simulink model "M37_Sim_Forcing_003h_expe_infra_transz_lim"  (Simulink 7.4)
settings: Solver=FixedStepDiscrete  StartTime=0.0  StopTime=inf  FixedStep=0.004  RelTol=1e-3
undefined symbols (not defined in the file or in its folder): DiscIntNeverNeededParam
libraries: simulink x39, gt_rt_lib x20, xpcutilitieslib x3, xpclib x2, dspswit3 x1
(part 3 of 4)

== system M37_Sim_Forcing_003h_expe_infra_transz_lim/Breaking_Control 20/07/15/Move_cabin/Subsystem ==
  com_or : Inport
  start_zeroing : Inport  Port=2
  connect_x : Inport  Port=3
  connect_z : Inport  Port=4
  reinit_ok : Inport  Port=5
  Display4 : Display
  Display5 : Display
  Embedded MATLAB Function3 : Stateflow chart
  Fcn : Fcn  Expr=abs(u(1))+abs(u(2))+abs(u(3))
  Logical Operator : Logic  Inputs=3  AllPortsSameDT=off  OutDataTypeMode=boolean  LogicDataType=fixdt(0, 8)  OutDataTypeStr=boolean
  Logical Operator1 : Logic  Operator=OR  AllPortsSameDT=off  OutDataTypeMode=boolean  LogicDataType=fixdt(0, 8)  OutDataTypeStr=boolean
  Logical Operator2 : Logic  Operator=NOT  AllPortsSameDT=off  OutDataTypeMode=boolean  LogicDataType=fixdt(0, 8)  OutDataTypeStr=boolean
  Logical Operator3 : Logic  AllPortsSameDT=off  OutDataTypeMode=boolean  LogicDataType=fixdt(0, 8)  OutDataTypeStr=boolean
  Logical Operator4 : Logic  AllPortsSameDT=off  OutDataTypeMode=boolean  LogicDataType=fixdt(0, 8)  OutDataTypeStr=boolean
  Logical Operator5 : Logic  Operator=OR  AllPortsSameDT=off  OutDataTypeMode=boolean  LogicDataType=fixdt(0, 8)  OutDataTypeStr=boolean
  Logical Operator6 : Logic  Operator=NOT  AllPortsSameDT=off  OutDataTypeMode=boolean  LogicDataType=fixdt(0, 8)  OutDataTypeStr=boolean
  Logical Operator7 : Logic  Inputs=4  AllPortsSameDT=off  OutDataTypeMode=boolean  LogicDataType=fixdt(0, 8)  OutDataTypeStr=boolean
  Logical Operator8 : Logic  Operator=NOT  Inputs=3  AllPortsSameDT=off  OutDataTypeMode=boolean  LogicDataType=fixdt(0, 8)  OutDataTypeStr=boolean
  Relational Operator : RelationalOperator  Operator=<=  LogicOutDataTypeMode=boolean  LogicDataType=fixdt(0, 8)  OutDataTypeStr=boolean
  Unit Delay : UnitDelay  SampleTime=-1
  gain : Constant  Value=0.004
  flag_reset : Outport  OutDataType=fixdt(1, 16)  OutScaling=2^0
  launch_reinit : Outport  Port=2  OutDataType=fixdt(1, 16)  OutScaling=2^0
  wires:
  gain/1 -> Relational Operator/2
  Logical Operator/1 -> Display4/1, flag_reset/1, Logical Operator8/1
  com_or/1 -> Embedded MATLAB Function3/1(com_or), Fcn/1
  Embedded MATLAB Function3/1(max_tilt) -> Relational Operator/1
  start_zeroing/1 -> Logical Operator3/1, Logical Operator5/1
  connect_x/1 -> Logical Operator3/2, Logical Operator6/1, Logical Operator7/3
  connect_z/1 -> Logical Operator2/1
  Logical Operator2/1 -> Logical Operator1/2
  Logical Operator3/1 -> Logical Operator1/1
  Logical Operator1/1 -> Logical Operator/2, Logical Operator7/2
  Relational Operator/1 -> Logical Operator4/1
  Logical Operator4/1 -> Logical Operator/1, Logical Operator7/1
  Logical Operator5/1 -> Logical Operator4/2
  Logical Operator6/1 -> Logical Operator5/2
  reinit_ok/1 -> Logical Operator/3
  Logical Operator7/1 -> launch_reinit/1, Display5/1
  Logical Operator8/1 -> Unit Delay/1
  Unit Delay/1 -> Logical Operator7/4

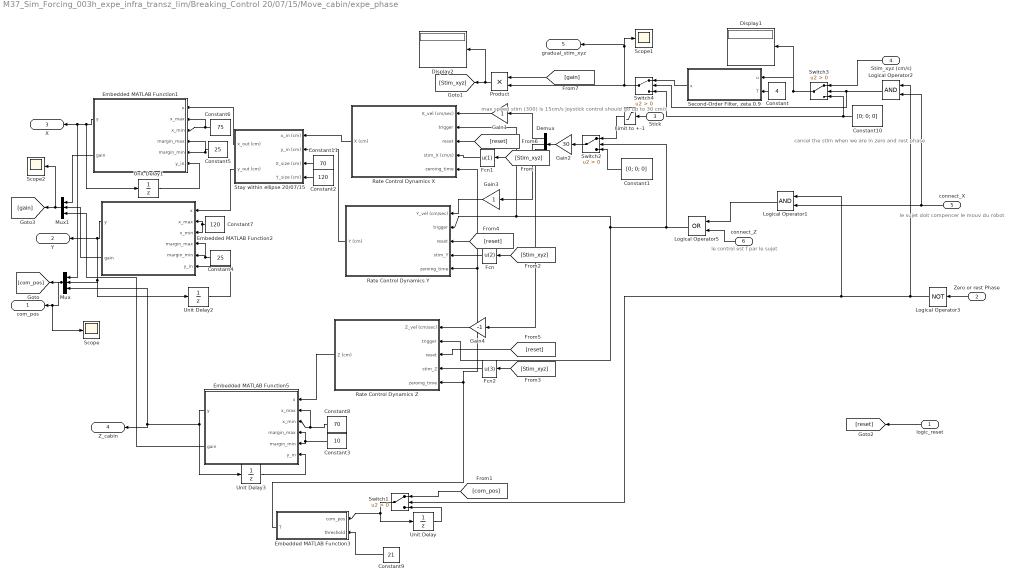
== system M37_Sim_Forcing_003h_expe_infra_transz_lim/Breaking_Control 20/07/15/Move_cabin/expe_phase ==
  note: cancel the stim when we are
      | in zero and rest phase
  note: max speed stim (300)
      | is 15cm/s
      | joystick control should go
      |  up to 30 cm/s
  note: le sujet doit compencer le mouv du robot
  note: le control est f par le sujet
  logic_reset : Inport
  Zero or rest Phase : Inport  Port=2  OutDataType=fixdt(1, 16)  OutScaling=2^0
  Stick : Inport  Port=3
  Stim_xyz (cm/s) : Inport  Port=4
  connect_X : Inport  Port=5  OutDataType=fixdt(1, 16)  OutScaling=2^0
  connect_Z : Inport  Port=6  OutDataType=fixdt(1, 16)  OutScaling=2^0
  Constant : Constant  Value=4  OutDataType=fixdt(1, 16)  OutScaling=2^0
  Constant1 : Constant  Value=[0; 0; 0]  OutDataType=fixdt(1, 16)  OutScaling=2^0
  Constant10 : Constant  Value=[0; 0; 0]  OutDataType=fixdt(1, 16)  OutScaling=2^0
  Constant11 : Constant  Value=70  OutDataType=fixdt(1, 16)  OutScaling=2^0
  Constant2 : Constant  Value=120  OutDataType=fixdt(1, 16)  OutScaling=2^0
  Constant3 : Constant  Value=10  OutDataType=fixdt(1, 16)  OutScaling=2^0
  Constant4 : Constant  Value=25  OutDataType=fixdt(1, 16)  OutScaling=2^0
  Constant5 : Constant  Value=25  OutDataType=fixdt(1, 16)  OutScaling=2^0
  Constant6 : Constant  Value=75  OutDataType=fixdt(1, 16)  OutScaling=2^0
  Constant7 : Constant  Value=120  OutDataType=fixdt(1, 16)  OutScaling=2^0
  Constant8 : Constant  Value=70  OutDataType=fixdt(1, 16)  OutScaling=2^0
  Constant9 : Constant  Value=21  OutDataType=fixdt(1, 16)  OutScaling=2^0
  Demux : Demux  Outputs=3
  Display1 : Display
  Display2 : Display
  Embedded MATLAB Function1 : Stateflow chart
  Embedded MATLAB Function2 : Stateflow chart
  Embedded MATLAB Function3 : Stateflow chart
  Embedded MATLAB Function5 : Stateflow chart
  Fcn : Fcn  Expr=u(2)
  Fcn1 : Fcn  Expr=u(1)
  Fcn2 : Fcn  Expr=u(3)
  Gain1 : Gain  ParameterDataType=fixdt(1, 16)  ParameterScaling=2^0  OutDataType=fixdt(1, 16)  OutScaling=2^0
  Gain2 : Gain  Gain=30  ParameterDataType=fixdt(1, 16)  ParameterScaling=2^0  OutDataType=fixdt(1, 16)  OutScaling=2^0
  Gain3 : Gain  ParameterDataType=fixdt(1, 16)  ParameterScaling=2^0  OutDataType=fixdt(1, 16)  OutScaling=2^0
  Gain4 : Gain  Gain=-1  ParameterDataType=fixdt(1, 16)  ParameterScaling=2^0  OutDataType=fixdt(1, 16)  OutScaling=2^0
  Limit to +-1 : Saturate  UpperLimit=1  LowerLimit=-1  OutDataType=fixdt(1, 16)  OutScaling=2^0
  Logical Operator1 : Logic  AllPortsSameDT=off  OutDataTypeMode=boolean  LogicDataType=fixdt(0, 8)  OutDataTypeStr=boolean
  Logical Operator2 : Logic  AllPortsSameDT=off  OutDataTypeMode=boolean  LogicDataType=fixdt(0, 8)  OutDataTypeStr=boolean
  Logical Operator3 : Logic  Operator=NOT  AllPortsSameDT=off  OutDataTypeMode=boolean  LogicDataType=fixdt(0, 8)  OutDataTypeStr=boolean
  Logical Operator5 : Logic  Operator=OR  AllPortsSameDT=off  OutDataTypeMode=boolean  LogicDataType=fixdt(0, 8)  OutDataTypeStr=boolean
  Mux : Mux  Inputs=3
  Mux1 : Mux  Inputs=3
  Product : Product  OutDataType=fixdt(1, 16)  OutScaling=2^0  RndMeth=Zero
  Rate Control Dynamics X : Subsystem
  Rate Control Dynamics Y : Subsystem
  Rate Control Dynamics Z : Subsystem
  Scope : Scope
      settings: TimeRange=10  YMax=65
  Scope1 : Scope
      settings: YMin=-0.5  YMax=10.5
  Scope2 : Scope
      settings: YMin=0.15  YMax=1  SaveName=ScopeData2
  "Second-Order Filter, zeta 0.9" : Subsystem
  Stay within ellipse 20/07/15 : Subsystem
  Switch{1..4} (4 alike) : Switch  Criteria=u2 > Threshold  OutDataType=fixdt(1, 16)  OutScaling=2^0
  Unit Delay : UnitDelay  X0=[0 0 0]  SampleTime=-1
  Unit Delay1 : UnitDelay  SampleTime=-1
  Unit Delay2 : UnitDelay  SampleTime=-1
  Unit Delay3 : UnitDelay  SampleTime=-1
  com_pos : Outport
  Y : Outport  Port=2
  X : Outport  Port=3
  Z_cabin : Outport  Port=4
  gradual_stim_xyz : Outport  Port=5
  wires:
  Gain2/1 -> Demux/1
  Demux/1 -> Gain1/1
  Demux/2 -> Gain3/1
  Switch2/1 -> Gain2/1
  Stick/1 -> Limit to +-1/1
  Demux/3 -> Gain4/1
  Zero or rest Phase/1 -> Logical Operator3/1
  Embedded MATLAB Function1/1(y) -> X/1, Mux/1, Unit Delay1/1
  Constant7/1 -> Embedded MATLAB Function2/2(x_max), Embedded MATLAB Function2/3(x_min)
  Embedded MATLAB Function2/1(y) -> Y/1, Mux/2, Unit Delay2/1
  Constant3/1 -> Embedded MATLAB Function5/5(margin_min), Embedded MATLAB Function5/4(margin_max)
  Constant8/1 -> Embedded MATLAB Function5/2(x_max), Embedded MATLAB Function5/3(x_min)
  Constant4/1 -> Embedded MATLAB Function2/4(margin_max), Embedded MATLAB Function2/5(margin_min)
  Constant5/1 -> Embedded MATLAB Function1/4(margin_max), Embedded MATLAB Function1/5(margin_min)
  Constant6/1 -> Embedded MATLAB Function1/3(x_min), Embedded MATLAB Function1/2(x_max)
  Constant9/1 -> Embedded MATLAB Function3/2(threshold)
  Switch1/1 -> Embedded MATLAB Function3/1(com_pos), Unit Delay/1
  Unit Delay/1 -> Switch1/3
  Embedded MATLAB Function3/1(T) -> Rate Control Dynamics X/5(zeroing_time), Rate Control Dynamics Y/5(zeroing_time), Rate Control Dynamics Z/5(zeroing_time)
  Mux/1 -> [com_pos], com_pos/1, Scope/1
  [com_pos] -> Switch1/1
  Gain3/1 -> Rate Control Dynamics Y/1(Y_vel (cm/sec))
  Gain4/1 -> Rate Control Dynamics Z/1(Z_vel (cm/sec))
  [Stim_xyz] -> Fcn/1
  [Stim_xyz] -> Fcn1/1
  [Stim_xyz] -> Fcn2/1
  Logical Operator3/1 -> Logical Operator2/1, Logical Operator1/1, Switch1/2
  Logical Operator1/1 -> Logical Operator5/1
  Constant1/1 -> Switch2/3
  Limit to +-1/1 -> Switch2/1
  connect_X/1 -> Logical Operator1/2, Logical Operator2/2
  Constant10/1 -> Switch3/3, Switch4/3
  Logical Operator2/1 -> Switch3/2, Switch4/2
  Switch3/1 -> Display1/1, "Second-Order Filter, zeta 0.9"/1(u)
  Stim_xyz (cm/s)/1 -> Switch3/1
  logic_reset/1 -> [reset]
  [reset] -> Rate Control Dynamics Y/3(reset)
  [reset] -> Rate Control Dynamics Z/3(reset)
  [reset] -> Rate Control Dynamics X/3(reset)
  Gain1/1 -> Rate Control Dynamics X/1(X_vel (cm/sec))
  Fcn1/1 -> Rate Control Dynamics X/4(stim_X (cm/s))
  Fcn/1 -> Rate Control Dynamics Y/4(stim_Y)
  Logical Operator5/1 -> Rate Control Dynamics Y/2(trigger), Rate Control Dynamics X/2(trigger), Rate Control Dynamics Z/2(trigger), Switch2/2
  connect_Z/1 -> Logical Operator5/2
  Rate Control Dynamics Z/1(Z (cm)) -> Embedded MATLAB Function5/1(x)
  Fcn2/1 -> Rate Control Dynamics Z/4(stim_Z)
  Stay within ellipse 20/07/15/1(x_out (cm)) -> Embedded MATLAB Function1/1(x)
  Stay within ellipse 20/07/15/2(y_out (cm)) -> Embedded MATLAB Function2/1(x)
  Rate Control Dynamics X/1(X (cm)) -> Stay within ellipse 20/07/15/1(x_in (cm))
  Rate Control Dynamics Y/1(Y (cm)) -> Stay within ellipse 20/07/15/2(y_in (cm))
  Constant2/1 -> Stay within ellipse 20/07/15/4(Y_size (cm))
  Constant11/1 -> Stay within ellipse 20/07/15/3(X_size (cm))
  Constant/1 -> "Second-Order Filter, zeta 0.9"/2(T)
  Switch4/1 -> gradual_stim_xyz/1, Scope1/1, Product/2
  "Second-Order Filter, zeta 0.9"/1(x) -> Switch4/1
  Unit Delay1/1 -> Embedded MATLAB Function1/6(y_in)
  Embedded MATLAB Function1/2(gain) -> Mux1/1
  Embedded MATLAB Function2/2(gain) -> Mux1/2
  Unit Delay2/1 -> Embedded MATLAB Function2/6(y_in)
  Embedded MATLAB Function5/1(y) -> Z_cabin/1, Mux/3, Unit Delay3/1
  Embedded MATLAB Function5/2(gain) -> Mux1/3
  Product/1 -> [Stim_xyz], Display2/1
  Mux1/1 -> [gain], Scope2/1
  [gain] -> Product/1
  Unit Delay3/1 -> Embedded MATLAB Function5/6(y_in)

== system M37_Sim_Forcing_003h_expe_infra_transz_lim/Breaking_Control 20/07/15/compute_offset/Smooth Displacement Second-Order Filter, zeta 0.8 ==
  Step IN Reset on  either : Inport
  T : Inport  Port=2  OutDataType=fixdt(1, 16)  OutScaling=2^0
  (zeta*T_transfer)/pi : Gain  Gain=0.8/pi  ParameterDataType=fixdt(1, 16)  ParameterScaling=2^0  OutDataType=fixdt(1, 16)  OutScaling=2^0
  4*zeta*pi : Gain  Gain=3.2*pi  ParameterDataType=fixdt(1, 16)  ParameterScaling=2^0  OutDataType=fixdt(1, 16)  OutScaling=2^0
  4*zeta*pi/T_transfer /s : DiscreteIntegrator  gainval=1  ExternalReset=either  InitialConditionSource=external  SampleTime=0.004  OutDataType=fixdt(1, 16)  OutScaling=2^0  ICPrevOutput=DiscIntNeverNeededParam  ICPrevScaledInput=DiscIntNeverNeededParam
  Discrete Derivative : simulink/Discrete/Discrete Derivative  SystemSampleTime=-1  gainval=1.0  ICPrevScaledInput=0.0  OutMin=[]  OutMax=[]  OutDataType=fixdt(1, 16)  OutScaling=2^-10  DoSatur=off
  Divide : Product  Inputs=*/  OutDataType=fixdt(1, 16)  OutScaling=2^-10
  Divide1 : Product  Inputs=*/  OutDataType=fixdt(1, 16)  OutScaling=2^-10
  For saving position  and velocity until after switchover : UnitDelay  SampleTime=-1
  Product : Product  OutDataType=fixdt(1, 16)  OutScaling=2^0  RndMeth=Zero
  Sum1 : Sum  Inputs=|+-  OutDataType=fixdt(1, 16)  OutScaling=2^0
  Sum2 : Sum  Inputs=-+|  OutDataType=fixdt(1, 16)  OutScaling=2^0
  pi/(zeta*T_transfer)/s : DiscreteIntegrator  gainval=1  ExternalReset=either  InitialConditionSource=external  SampleTime=0.004  OutDataType=fixdt(1, 16)  OutScaling=2^0  ICPrevOutput=DiscIntNeverNeededParam  ICPrevScaledInput=DiscIntNeverNeededParam
  pi/zeta : Gain  Gain=pi/0.8  ParameterDataType=fixdt(1, 16)  ParameterScaling=2^0  OutDataType=fixdt(1, 16)  OutScaling=2^0
  Out : Outport
  wires:
  Discrete Derivative/1 -> Product/2
  Product/1 -> (zeta*T_transfer)/pi/1
  Divide/1 -> 4*zeta*pi/1
  Divide1/1 -> pi/zeta/1
  pi/zeta/1 -> pi/(zeta*T_transfer)/s/1
  pi/(zeta*T_transfer)/s/1 -> Sum2/1, Out/1, For saving position  and velocity until after switchover/1
  4*zeta*pi/T_transfer /s/1 -> Divide1/1, Sum1/2
  Sum1/1 -> Divide/1
  4*zeta*pi/1 -> 4*zeta*pi/T_transfer /s/1
  T/1 -> [T]
  Step IN Reset on  either/1 -> [Step], Sum2/2
  [Step] -> 4*zeta*pi/T_transfer /s/2
  [Step] -> pi/(zeta*T_transfer)/s/2
  [T] -> Divide/2
  For saving position  and velocity until after switchover/1 -> Discrete Derivative/1, pi/(zeta*T_transfer)/s/3
  [T] -> Product/1
  (zeta*T_transfer)/pi/1 -> 4*zeta*pi/T_transfer /s/3
  [T] -> Divide1/2
  Sum2/1 -> Sum1/1

== system M37_Sim_Forcing_003h_expe_infra_transz_lim/Joint Controller (May 7, 2015)1/Forward Kinematics/KUKA2NED ==
  KUKA : Inport
  Constant : Constant  Value=[0 0 0 0 0 15.89]  OutDataType=fixdt(1, 16)  OutScaling=2^0
  Gain : Gain  Gain=[1 -1 -1 -1 -1 -1]  ParameterDataType=fixdt(1, 16)  ParameterScaling=2^0  OutDataType=fixdt(1, 16)  OutScaling=2^0
  Sum : Sum  Inputs=|++  OutDataType=fixdt(1, 16)  OutScaling=2^0
  NED : Outport
  wires:
  Gain/1 -> Sum/1
  KUKA/1 -> Gain/1
  Sum/1 -> NED/1
  Constant/1 -> Sum/2

== system M37_Sim_Forcing_003h_expe_infra_transz_lim/Joint Controller (May 7, 2015)1/Inverse Kinematics May 6, 2015/Inverse Kinematics ==
  note: (6_DOF_ACT - 6_DOF_COM) exp(-0.1t) + 6_DOF_COM
  vec : Inport
  Activate full inverse : Inport  Port=2
  6_DOF_ACT : Inport  Port=3  OutDataType=fixdt(1, 16)  OutScaling=2^0
  Demux : Demux  Outputs=[6,6]
  Discrete-Time Integrator : DiscreteIntegrator  gainval=1  ExternalReset=either  InitialConditionSource=external  SampleTime=-1  OutDataType=fixdt(1, 16)  OutScaling=2^0  ICPrevOutput=DiscIntNeverNeededParam  ICPrevScaledInput=DiscIntNeverNeededParam
  Gain : Gain  Gain=-0.1  ParameterDataType=fixdt(1, 16)  ParameterScaling=2^0  OutDataType=fixdt(1, 16)  OutScaling=2^0
  Mux : Mux  Inputs=2
  Select -6_DOF_COM : Selector  InputPortWidth=12  IndexOptions=Index vector (dialog)  Indices=[1 2 3 4 5 6]  OutputSizes=1
  Sum : Sum  Inputs=|-+  OutDataType=fixdt(1, 16)  OutScaling=2^0
  Sum1 : Sum  Inputs=|++  OutDataType=fixdt(1, 16)  OutScaling=2^0
  full inverse kin : Subsystem
  out : Outport  OutDataType=fixdt(1, 16)  OutScaling=2^0
  wires:
  vec/1 -> Select -6_DOF_COM/1, Demux/1
  full inverse kin/1(out) -> out/1
  Activate full inverse/1 -> full inverse kin/Enable, Discrete-Time Integrator/2
  Discrete-Time Integrator/1 -> Gain/1, Sum1/2
  Gain/1 -> Discrete-Time Integrator/1
  6_DOF_ACT/1 -> Sum/2
  Select -6_DOF_COM/1 -> Sum/1
  Sum/1 -> Discrete-Time Integrator/3
  Demux/2 -> Mux/2
  Demux/1 -> Sum1/1
  Sum1/1 -> Mux/1
  Mux/1 -> full inverse kin/1(vec)

== system M37_Sim_Forcing_003h_expe_infra_transz_lim/Joint Controller (May 7, 2015)1/Inverse Kinematics May 6, 2015/NED2KUKA ==
  NED : Inport
  Constant : Constant  Value=[0 0 0 0 0 15.89]  OutDataType=fixdt(1, 16)  OutScaling=2^0
  Gain : Gain  Gain=[1 -1 -1 -1 -1 -1]  ParameterDataType=fixdt(1, 16)  ParameterScaling=2^0  OutDataType=fixdt(1, 16)  OutScaling=2^0
  Sum : Sum  Inputs=|++  OutDataType=fixdt(1, 16)  OutScaling=2^0
  KUKA : Outport
  wires:
  Gain/1 -> Sum/1
  NED/1 -> Gain/1
  Sum/1 -> KUKA/1
  Constant/1 -> Sum/2

== system M37_Sim_Forcing_003h_expe_infra_transz_lim/Joint Controller (May 7, 2015)1/Inverse Kinematics May 6, 2015/Simplified Inverse Kinematics ==
  note: (A1-A6_ACT - A1-A6_COM) exp(-0.1t) + A1-A6_COM
  note: Selects and sets
      |  A1, A4,A6 to zero
  note: This version has been tested on May 6, 2015
  activate simplified : Inport  OutDataType=fixdt(1, 16)  OutScaling=2^0
  vec : Inport  Port=2  OutDataType=fixdt(1, 16)  OutScaling=2^0
  A1-A6 ACT : Selector  InputPortWidth=12  IndexOptions=Index vector (dialog)  Indices=[7 8 9 10 11 12]  OutputSizes=1
  A1-A6 COM : Subsystem
  Discrete-Time Integrator1 : DiscreteIntegrator  gainval=1  ExternalReset=either  InitialConditionSource=external  SampleTime=-1  OutDataType=fixdt(1, 16)  OutScaling=2^0  ICPrevOutput=DiscIntNeverNeededParam  ICPrevScaledInput=DiscIntNeverNeededParam
  Gain1 : Gain  Gain=-0.1  ParameterDataType=fixdt(1, 16)  ParameterScaling=2^0  OutDataType=fixdt(1, 16)  OutScaling=2^0
  Mux : Mux  Inputs=2
  N : Selector  InputPortWidth=7  IndexOptions=Index vector (dialog)  Indices=7  OutputSizes=1
  Simplified Inverse Kin : Subsystem
  Sum : Sum  Inputs=-+|  OutDataType=fixdt(1, 16)  OutScaling=2^0
  Sum1 : Sum  Inputs=++|  OutDataType=fixdt(1, 16)  OutScaling=2^0
  out : Outport  OutDataType=fixdt(1, 16)  OutScaling=2^0
  outMGI : Outport  Port=2  OutDataType=fixdt(1, 16)  OutScaling=2^0
  wires:
  vec/1 -> Simplified Inverse Kin/1(Vec), A1-A6 ACT/1
  activate simplified/1 -> Simplified Inverse Kin/Enable, Discrete-Time Integrator1/2
  Discrete-Time Integrator1/1 -> Gain1/1, Sum1/2
  Gain1/1 -> Discrete-Time Integrator1/1
  Sum1/1 -> Mux/1
  Sum/1 -> Discrete-Time Integrator1/3
  Mux/1 -> out/1
  A1-A6 ACT/1 -> Sum/2
  Simplified Inverse Kin/1(Out) -> A1-A6 COM/1(vec), N/1
  A1-A6 COM/1(A1-A6 COM) -> Sum/1, Sum1/1
  N/1 -> Mux/2
  Simplified Inverse Kin/2(Out_MGI) -> outMGI/1

== system M37_Sim_Forcing_003h_expe_infra_transz_lim/BEC (May 7, 2015)/CAN Send/If Action Subsystem1/Convert int to 4*uni8  ==
  in : Inport
  Gain{1..4} (4 alike) : Gain  ParameterDataType=fixdt(1, 16)  ParameterScaling=2^0  OutDataTypeMode=uint8  OutDataType=fixdt(1, 16)  OutScaling=2^0  OutDataTypeStr=uint8
  Mux : Mux
  Shift Arithmetic : simulink/Logic and Bit Operations/Shift Arithmetic  SystemSampleTime=-1  nBitShiftRight=8  nBinPtShiftRight=0
  Shift Arithmetic1 : simulink/Logic and Bit Operations/Shift Arithmetic  SystemSampleTime=-1  nBitShiftRight=16  nBinPtShiftRight=0
  Shift Arithmetic2 : simulink/Logic and Bit Operations/Shift Arithmetic  SystemSampleTime=-1  nBitShiftRight=24  nBinPtShiftRight=0
  out : Outport
  wires:
  in/1 -> Shift Arithmetic1/1, Gain1/1, Shift Arithmetic/1, Shift Arithmetic2/1
  Shift Arithmetic/1 -> Gain2/1
  Shift Arithmetic1/1 -> Gain3/1
  Shift Arithmetic2/1 -> Gain4/1
  Gain1/1 -> Mux/1
  Gain2/1 -> Mux/2
  Gain3/1 -> Mux/3
  Gain4/1 -> Mux/4
  Mux/1 -> out/1

== system M37_Sim_Forcing_003h_expe_infra_transz_lim/BEC (May 7, 2015)/CAN Send/If Action Subsystem1/Convert int to 4*uni8 1 ==
  in : Inport
  Gain{1..4} (4 alike) : Gain  ParameterDataType=fixdt(1, 16)  ParameterScaling=2^0  OutDataTypeMode=uint8  OutDataType=fixdt(1, 16)  OutScaling=2^0  OutDataTypeStr=uint8
  Mux : Mux
  Shift Arithmetic : simulink/Logic and Bit Operations/Shift Arithmetic  SystemSampleTime=-1  nBitShiftRight=8  nBinPtShiftRight=0
  Shift Arithmetic1 : simulink/Logic and Bit Operations/Shift Arithmetic  SystemSampleTime=-1  nBitShiftRight=16  nBinPtShiftRight=0
  Shift Arithmetic2 : simulink/Logic and Bit Operations/Shift Arithmetic  SystemSampleTime=-1  nBitShiftRight=24  nBinPtShiftRight=0
  out : Outport
  wires:
  Mux/1 -> out/1
  Gain4/1 -> Mux/4
  Gain3/1 -> Mux/3
  Gain2/1 -> Mux/2
  Gain1/1 -> Mux/1
  Shift Arithmetic2/1 -> Gain4/1
  Shift Arithmetic1/1 -> Gain3/1
  Shift Arithmetic/1 -> Gain2/1
  in/1 -> Shift Arithmetic2/1, Shift Arithmetic/1, Gain1/1, Shift Arithmetic1/1

== system M37_Sim_Forcing_003h_expe_infra_transz_lim/BEC (May 7, 2015)/CAN Send/If Action Subsystem1/Convert int to 4*uni8 2 ==
  in : Inport
  Gain{1..4} (4 alike) : Gain  ParameterDataType=fixdt(1, 16)  ParameterScaling=2^0  OutDataTypeMode=uint8  OutDataType=fixdt(1, 16)  OutScaling=2^0  OutDataTypeStr=uint8
  Mux : Mux
  Shift Arithmetic : simulink/Logic and Bit Operations/Shift Arithmetic  SystemSampleTime=-1  nBitShiftRight=8  nBinPtShiftRight=0
  Shift Arithmetic1 : simulink/Logic and Bit Operations/Shift Arithmetic  SystemSampleTime=-1  nBitShiftRight=16  nBinPtShiftRight=0
  Shift Arithmetic2 : simulink/Logic and Bit Operations/Shift Arithmetic  SystemSampleTime=-1  nBitShiftRight=24  nBinPtShiftRight=0
  out : Outport
  wires:
  Mux/1 -> out/1
  Gain4/1 -> Mux/4
  Gain3/1 -> Mux/3
  Gain2/1 -> Mux/2
  Gain1/1 -> Mux/1
  Shift Arithmetic2/1 -> Gain4/1
  Shift Arithmetic1/1 -> Gain3/1
  Shift Arithmetic/1 -> Gain2/1
  in/1 -> Shift Arithmetic2/1, Shift Arithmetic/1, Gain1/1, Shift Arithmetic1/1

== system M37_Sim_Forcing_003h_expe_infra_transz_lim/BEC (May 7, 2015)/CAN Send/If Action Subsystem1/Convert int to 4*uni8 3 ==
  in : Inport
  Gain{1..4} (4 alike) : Gain  ParameterDataType=fixdt(1, 16)  ParameterScaling=2^0  OutDataTypeMode=uint8  OutDataType=fixdt(1, 16)  OutScaling=2^0  OutDataTypeStr=uint8
  Mux : Mux
  Shift Arithmetic : simulink/Logic and Bit Operations/Shift Arithmetic  SystemSampleTime=-1  nBitShiftRight=8  nBinPtShiftRight=0
  Shift Arithmetic1 : simulink/Logic and Bit Operations/Shift Arithmetic  SystemSampleTime=-1  nBitShiftRight=16  nBinPtShiftRight=0
  Shift Arithmetic2 : simulink/Logic and Bit Operations/Shift Arithmetic  SystemSampleTime=-1  nBitShiftRight=24  nBinPtShiftRight=0
  out : Outport
  wires:
  in/1 -> Shift Arithmetic1/1, Gain1/1, Shift Arithmetic/1, Shift Arithmetic2/1
  Shift Arithmetic/1 -> Gain2/1
  Shift Arithmetic1/1 -> Gain3/1
  Shift Arithmetic2/1 -> Gain4/1
  Gain1/1 -> Mux/1
  Gain2/1 -> Mux/2
  Gain3/1 -> Mux/3
  Gain4/1 -> Mux/4
  Mux/1 -> out/1

== system M37_Sim_Forcing_003h_expe_infra_transz_lim/BEC (May 7, 2015)/CAN Send/If Action Subsystem1/Convert int to 4*uni8 4 ==
  in : Inport
  Gain{1..4} (4 alike) : Gain  ParameterDataType=fixdt(1, 16)  ParameterScaling=2^0  OutDataTypeMode=uint8  OutDataType=fixdt(1, 16)  OutScaling=2^0  OutDataTypeStr=uint8
  Mux : Mux
  Shift Arithmetic : simulink/Logic and Bit Operations/Shift Arithmetic  SystemSampleTime=-1  nBitShiftRight=8  nBinPtShiftRight=0
  Shift Arithmetic1 : simulink/Logic and Bit Operations/Shift Arithmetic  SystemSampleTime=-1  nBitShiftRight=16  nBinPtShiftRight=0
  Shift Arithmetic2 : simulink/Logic and Bit Operations/Shift Arithmetic  SystemSampleTime=-1  nBitShiftRight=24  nBinPtShiftRight=0
  out : Outport
  wires:
  in/1 -> Shift Arithmetic1/1, Gain1/1, Shift Arithmetic/1, Shift Arithmetic2/1
  Shift Arithmetic/1 -> Gain2/1
  Shift Arithmetic1/1 -> Gain3/1
  Shift Arithmetic2/1 -> Gain4/1
  Gain1/1 -> Mux/1
  Gain2/1 -> Mux/2
  Gain3/1 -> Mux/3
  Gain4/1 -> Mux/4
  Mux/1 -> out/1

== system M37_Sim_Forcing_003h_expe_infra_transz_lim/BEC (May 7, 2015)/CAN Send/If Action Subsystem1/Convert int to 4*uni8 5 ==
  in : Inport
  Gain{1..4} (4 alike) : Gain  ParameterDataType=fixdt(1, 16)  ParameterScaling=2^0  OutDataTypeMode=uint8  OutDataType=fixdt(1, 16)  OutScaling=2^0  OutDataTypeStr=uint8
  Mux : Mux
  Shift Arithmetic : simulink/Logic and Bit Operations/Shift Arithmetic  SystemSampleTime=-1  nBitShiftRight=8  nBinPtShiftRight=0
  Shift Arithmetic1 : simulink/Logic and Bit Operations/Shift Arithmetic  SystemSampleTime=-1  nBitShiftRight=16  nBinPtShiftRight=0
  Shift Arithmetic2 : simulink/Logic and Bit Operations/Shift Arithmetic  SystemSampleTime=-1  nBitShiftRight=24  nBinPtShiftRight=0
  out : Outport
  wires:
  Mux/1 -> out/1
  Gain4/1 -> Mux/4
  Gain3/1 -> Mux/3
  Gain2/1 -> Mux/2
  Gain1/1 -> Mux/1
  Shift Arithmetic2/1 -> Gain4/1
  Shift Arithmetic1/1 -> Gain3/1
  Shift Arithmetic/1 -> Gain2/1
  in/1 -> Shift Arithmetic2/1, Shift Arithmetic/1, Gain1/1, Shift Arithmetic1/1

== system M37_Sim_Forcing_003h_expe_infra_transz_lim/BEC (May 7, 2015)/Software limit switches/Subsystem/If Action Subsystem ==
  dif : Inport  OutDataType=fixdt(1, 16)  OutScaling=2^0
  Inc : Inport  Port=2  OutDataType=fixdt(1, 16)  OutScaling=2^0
  Action Port : ActionPort  ActionType=then
  PSEA2 : Constant  Value=0  OutDataType=fixdt(1, 16)  OutScaling=2^0
  Switch : Switch  Criteria=u2 > Threshold  Threshold=1  OutDataType=fixdt(1, 16)  OutScaling=2^0
  Out1 : Outport  OutDataType=fixdt(1, 16)  OutScaling=2^0
  wires:
  PSEA2/1 -> Switch/3
  Switch/1 -> Out1/1
  Inc/1 -> Switch/1
  dif/1 -> Switch/2

== system M37_Sim_Forcing_003h_expe_infra_transz_lim/BEC (May 7, 2015)/Software limit switches/Subsystem/If Action Subsystem1 ==
  Inc : Inport  OutDataType=fixdt(1, 16)  OutScaling=2^0
  dif : Inport  Port=2  OutDataType=fixdt(1, 16)  OutScaling=2^0
  Action Port : ActionPort  ActionType=else
  PSEA2 : Constant  Value=0  OutDataType=fixdt(1, 16)  OutScaling=2^0
  Switch : Switch  Threshold=1  OutDataType=fixdt(1, 16)  OutScaling=2^0
  Out1 : Outport  OutDataType=fixdt(1, 16)  OutScaling=2^0
  wires:
  dif/1 -> Switch/2
  Inc/1 -> Switch/1
  Switch/1 -> Out1/1
  PSEA2/1 -> Switch/3

== system M37_Sim_Forcing_003h_expe_infra_transz_lim/BEC (May 7, 2015)/Software limit switches/Subsystem1/If Action Subsystem ==
  dif : Inport  OutDataType=fixdt(1, 16)  OutScaling=2^0
  Inc : Inport  Port=2  OutDataType=fixdt(1, 16)  OutScaling=2^0
  Action Port : ActionPort  ActionType=then
  PSEA2 : Constant  Value=0  OutDataType=fixdt(1, 16)  OutScaling=2^0
  Switch : Switch  Threshold=1  OutDataType=fixdt(1, 16)  OutScaling=2^0
  Out1 : Outport  OutDataType=fixdt(1, 16)  OutScaling=2^0
  wires:
  dif/1 -> Switch/2
  Inc/1 -> Switch/1
  Switch/1 -> Out1/1
  PSEA2/1 -> Switch/3

== system M37_Sim_Forcing_003h_expe_infra_transz_lim/BEC (May 7, 2015)/Software limit switches/Subsystem1/If Action Subsystem1 ==
  Inc : Inport  OutDataType=fixdt(1, 16)  OutScaling=2^0
  dif : Inport  Port=2  OutDataType=fixdt(1, 16)  OutScaling=2^0
  Action Port : ActionPort  ActionType=else
  PSEA2 : Constant  Value=0  OutDataType=fixdt(1, 16)  OutScaling=2^0
  Switch : Switch  Threshold=1  OutDataType=fixdt(1, 16)  OutScaling=2^0
  Out1 : Outport  OutDataType=fixdt(1, 16)  OutScaling=2^0
  wires:
  PSEA2/1 -> Switch/3
  Switch/1 -> Out1/1
  Inc/1 -> Switch/1
  dif/1 -> Switch/2

== system M37_Sim_Forcing_003h_expe_infra_transz_lim/BEC (May 7, 2015)/Software limit switches/Subsystem2/If Action Subsystem ==
  dif : Inport  OutDataType=fixdt(1, 16)  OutScaling=2^0
  Inc : Inport  Port=2  OutDataType=fixdt(1, 16)  OutScaling=2^0
  Action Port : ActionPort  ActionType=then
  PSEA2 : Constant  Value=0  OutDataType=fixdt(1, 16)  OutScaling=2^0
  Switch : Switch  Threshold=1  OutDataType=fixdt(1, 16)  OutScaling=2^0
  Out1 : Outport  OutDataType=fixdt(1, 16)  OutScaling=2^0
  wires:
  PSEA2/1 -> Switch/3
  Switch/1 -> Out1/1
  Inc/1 -> Switch/1
  dif/1 -> Switch/2

== system M37_Sim_Forcing_003h_expe_infra_transz_lim/BEC (May 7, 2015)/Software limit switches/Subsystem2/If Action Subsystem1 ==
  Inc : Inport  OutDataType=fixdt(1, 16)  OutScaling=2^0
  dif : Inport  Port=2  OutDataType=fixdt(1, 16)  OutScaling=2^0
  Action Port : ActionPort  ActionType=else
  PSEA2 : Constant  Value=0  OutDataType=fixdt(1, 16)  OutScaling=2^0
  Switch : Switch  Threshold=1  OutDataType=fixdt(1, 16)  OutScaling=2^0
  Out1 : Outport  OutDataType=fixdt(1, 16)  OutScaling=2^0
  wires:
  dif/1 -> Switch/2
  Inc/1 -> Switch/1
  Switch/1 -> Out1/1
  PSEA2/1 -> Switch/3

== system M37_Sim_Forcing_003h_expe_infra_transz_lim/BEC (May 7, 2015)/Software limit switches/Subsystem3/If Action Subsystem ==
  dif : Inport  OutDataType=fixdt(1, 16)  OutScaling=2^0
  Inc : Inport  Port=2  OutDataType=fixdt(1, 16)  OutScaling=2^0
  Action Port : ActionPort  ActionType=then
  PSEA2 : Constant  Value=0  OutDataType=fixdt(1, 16)  OutScaling=2^0
  Switch : Switch  Threshold=1  OutDataType=fixdt(1, 16)  OutScaling=2^0
  Out1 : Outport  OutDataType=fixdt(1, 16)  OutScaling=2^0
  wires:
  dif/1 -> Switch/2
  Inc/1 -> Switch/1
  Switch/1 -> Out1/1
  PSEA2/1 -> Switch/3

== system M37_Sim_Forcing_003h_expe_infra_transz_lim/BEC (May 7, 2015)/Software limit switches/Subsystem3/If Action Subsystem1 ==
  Inc : Inport  OutDataType=fixdt(1, 16)  OutScaling=2^0
  dif : Inport  Port=2  OutDataType=fixdt(1, 16)  OutScaling=2^0
  Action Port : ActionPort  ActionType=else
  PSEA2 : Constant  Value=0  OutDataType=fixdt(1, 16)  OutScaling=2^0
  Switch : Switch  Threshold=1  OutDataType=fixdt(1, 16)  OutScaling=2^0
  Out1 : Outport  OutDataType=fixdt(1, 16)  OutScaling=2^0
  wires:
  PSEA2/1 -> Switch/3
  Switch/1 -> Out1/1
  Inc/1 -> Switch/1
  dif/1 -> Switch/2

== system M37_Sim_Forcing_003h_expe_infra_transz_lim/BEC (May 7, 2015)/Software limit switches/Subsystem4/If Action Subsystem ==
  dif : Inport  OutDataType=fixdt(1, 16)  OutScaling=2^0
  Inc : Inport  Port=2  OutDataType=fixdt(1, 16)  OutScaling=2^0
  Action Port : ActionPort  ActionType=then
  PSEA2 : Constant  Value=0  OutDataType=fixdt(1, 16)  OutScaling=2^0
  Switch : Switch  Threshold=1  OutDataType=fixdt(1, 16)  OutScaling=2^0
  Out1 : Outport  OutDataType=fixdt(1, 16)  OutScaling=2^0
  wires:
  PSEA2/1 -> Switch/3
  Switch/1 -> Out1/1
  Inc/1 -> Switch/1
  dif/1 -> Switch/2

== system M37_Sim_Forcing_003h_expe_infra_transz_lim/BEC (May 7, 2015)/Software limit switches/Subsystem4/If Action Subsystem1 ==
  Inc : Inport  OutDataType=fixdt(1, 16)  OutScaling=2^0
  dif : Inport  Port=2  OutDataType=fixdt(1, 16)  OutScaling=2^0
  Action Port : ActionPort  ActionType=else
  PSEA2 : Constant  Value=0  OutDataType=fixdt(1, 16)  OutScaling=2^0
  Switch : Switch  Threshold=1  OutDataType=fixdt(1, 16)  OutScaling=2^0
  Out1 : Outport  OutDataType=fixdt(1, 16)  OutScaling=2^0
  wires:
  dif/1 -> Switch/2
  Inc/1 -> Switch/1
  Switch/1 -> Out1/1
  PSEA2/1 -> Switch/3

== system M37_Sim_Forcing_003h_expe_infra_transz_lim/BEC (May 7, 2015)/Software limit switches/Subsystem5/If Action Subsystem ==
  dif : Inport  OutDataType=fixdt(1, 16)  OutScaling=2^0
  Inc : Inport  Port=2  OutDataType=fixdt(1, 16)  OutScaling=2^0
  Action Port : ActionPort  ActionType=then
  PSEA2 : Constant  Value=0  OutDataType=fixdt(1, 16)  OutScaling=2^0
  Switch : Switch  Threshold=1  OutDataType=fixdt(1, 16)  OutScaling=2^0
  Out1 : Outport  OutDataType=fixdt(1, 16)  OutScaling=2^0
  wires:
  dif/1 -> Switch/2
  Inc/1 -> Switch/1
  Switch/1 -> Out1/1
  PSEA2/1 -> Switch/3

== system M37_Sim_Forcing_003h_expe_infra_transz_lim/BEC (May 7, 2015)/Software limit switches/Subsystem5/If Action Subsystem1 ==
  Inc : Inport  OutDataType=fixdt(1, 16)  OutScaling=2^0
  dif : Inport  Port=2  OutDataType=fixdt(1, 16)  OutScaling=2^0
  Action Port : ActionPort  ActionType=else
  PSEA2 : Constant  Value=0  OutDataType=fixdt(1, 16)  OutScaling=2^0
  Switch : Switch  Threshold=1  OutDataType=fixdt(1, 16)  OutScaling=2^0
  Out1 : Outport  OutDataType=fixdt(1, 16)  OutScaling=2^0
  wires:
  PSEA2/1 -> Switch/3
  Switch/1 -> Out1/1
  Inc/1 -> Switch/1
  dif/1 -> Switch/2

== system M37_Sim_Forcing_003h_expe_infra_transz_lim/Breaking_Control 20/07/15/Ellipse motion/Phase Shifted Sine 17th 1/Smooth Displacement Second-Order Filter, zeta 0.8 ==
  Step IN Reset on  either : Inport
  T : Inport  Port=2  OutDataType=fixdt(1, 16)  OutScaling=2^0
  (zeta*T_transfer)/pi : Gain  Gain=0.8/pi  ParameterDataType=fixdt(1, 16)  ParameterScaling=2^0  OutDataType=fixdt(1, 16)  OutScaling=2^0
  4*zeta*pi : Gain  Gain=3.2*pi  ParameterDataType=fixdt(1, 16)  ParameterScaling=2^0  OutDataType=fixdt(1, 16)  OutScaling=2^0
  4*zeta*pi/T_transfer /s : DiscreteIntegrator  gainval=1  ExternalReset=either  InitialConditionSource=external  SampleTime=-1  OutDataType=fixdt(1, 16)  OutScaling=2^0  ICPrevOutput=DiscIntNeverNeededParam  ICPrevScaledInput=DiscIntNeverNeededParam
  Data Type Conversion4 : DataTypeConversion  OutDataTypeMode=single  OutDataType=fixdt(1, 16)  OutScaling=2^0  OutDataTypeStr=single
  Discrete Derivative : simulink/Discrete/Discrete Derivative  SystemSampleTime=-1  gainval=1.0  ICPrevScaledInput=0.0  OutMin=[]  OutMax=[]  OutDataType=fixdt(1, 16)  OutScaling=2^-10  DoSatur=off
  Divide : Product  Inputs=*/  OutDataType=fixdt(1, 16)  OutScaling=2^-10
  Divide1 : Product  Inputs=*/  OutDataType=fixdt(1, 16)  OutScaling=2^-10
  For saving position  and velocity until after switchover : UnitDelay  SampleTime=-1
  Product : Product  OutDataType=fixdt(1, 16)  OutScaling=2^0  RndMeth=Zero
  Sum1 : Sum  Inputs=|+-  OutDataType=fixdt(1, 16)  OutScaling=2^0
  Sum2 : Sum  Inputs=-+|  OutDataType=fixdt(1, 16)  OutScaling=2^0
  pi/(zeta*T_transfer)/s : DiscreteIntegrator  gainval=1  ExternalReset=either  InitialConditionSource=external  SampleTime=-1  OutDataType=fixdt(1, 16)  OutScaling=2^0  ICPrevOutput=DiscIntNeverNeededParam  ICPrevScaledInput=DiscIntNeverNeededParam
  pi/zeta : Gain  Gain=pi/0.8  ParameterDataType=fixdt(1, 16)  ParameterScaling=2^0  OutDataType=fixdt(1, 16)  OutScaling=2^0
  Out : Outport
  wires:
  Discrete Derivative/1 -> Product/2
  Product/1 -> (zeta*T_transfer)/pi/1
  Divide/1 -> 4*zeta*pi/1
  Divide1/1 -> pi/zeta/1
  pi/zeta/1 -> pi/(zeta*T_transfer)/s/1
  pi/(zeta*T_transfer)/s/1 -> Sum2/1, For saving position  and velocity until after switchover/1, Data Type Conversion4/1
  4*zeta*pi/T_transfer /s/1 -> Divide1/1, Sum1/2
  Sum1/1 -> Divide/1
  4*zeta*pi/1 -> 4*zeta*pi/T_transfer /s/1
  T/1 -> [T]
  Step IN Reset on  either/1 -> [Step], Sum2/2
  [Step] -> 4*zeta*pi/T_transfer /s/2
  [Step] -> pi/(zeta*T_transfer)/s/2
  [T] -> Divide/2
  For saving position  and velocity until after switchover/1 -> Discrete Derivative/1, pi/(zeta*T_transfer)/s/3
  [T] -> Product/1
  (zeta*T_transfer)/pi/1 -> 4*zeta*pi/T_transfer /s/3
  [T] -> Divide1/2
  Sum2/1 -> Sum1/1
  Data Type Conversion4/1 -> Out/1

== system M37_Sim_Forcing_003h_expe_infra_transz_lim/Breaking_Control 20/07/15/Ellipse motion/Phase Shifted Sine 17th 2/Smooth Displacement Second-Order Filter, zeta 0.8 ==
  Step IN Reset on  either : Inport
  T : Inport  Port=2  OutDataType=fixdt(1, 16)  OutScaling=2^0
  (zeta*T_transfer)/pi : Gain  Gain=0.8/pi  ParameterDataType=fixdt(1, 16)  ParameterScaling=2^0  OutDataType=fixdt(1, 16)  OutScaling=2^0
  4*zeta*pi : Gain  Gain=3.2*pi  ParameterDataType=fixdt(1, 16)  ParameterScaling=2^0  OutDataType=fixdt(1, 16)  OutScaling=2^0
  4*zeta*pi/T_transfer /s : DiscreteIntegrator  gainval=1  ExternalReset=either  InitialConditionSource=external  SampleTime=-1  OutDataType=fixdt(1, 16)  OutScaling=2^0  ICPrevOutput=DiscIntNeverNeededParam  ICPrevScaledInput=DiscIntNeverNeededParam
  Data Type Conversion4 : DataTypeConversion  OutDataTypeMode=single  OutDataType=fixdt(1, 16)  OutScaling=2^0  OutDataTypeStr=single
  Discrete Derivative : simulink/Discrete/Discrete Derivative  SystemSampleTime=-1  gainval=1.0  ICPrevScaledInput=0.0  OutMin=[]  OutMax=[]  OutDataType=fixdt(1, 16)  OutScaling=2^-10  DoSatur=off
  Divide : Product  Inputs=*/  OutDataType=fixdt(1, 16)  OutScaling=2^-10
  Divide1 : Product  Inputs=*/  OutDataType=fixdt(1, 16)  OutScaling=2^-10
  For saving position  and velocity until after switchover : UnitDelay  SampleTime=-1
  Product : Product  OutDataType=fixdt(1, 16)  OutScaling=2^0  RndMeth=Zero
  Sum1 : Sum  Inputs=|+-  OutDataType=fixdt(1, 16)  OutScaling=2^0
  Sum2 : Sum  Inputs=-+|  OutDataType=fixdt(1, 16)  OutScaling=2^0
  pi/(zeta*T_transfer)/s : DiscreteIntegrator  gainval=1  ExternalReset=either  InitialConditionSource=external  SampleTime=-1  OutDataType=fixdt(1, 16)  OutScaling=2^0  ICPrevOutput=DiscIntNeverNeededParam  ICPrevScaledInput=DiscIntNeverNeededParam
  pi/zeta : Gain  Gain=pi/0.8  ParameterDataType=fixdt(1, 16)  ParameterScaling=2^0  OutDataType=fixdt(1, 16)  OutScaling=2^0
  Out : Outport
  wires:
  Discrete Derivative/1 -> Product/2
  Product/1 -> (zeta*T_transfer)/pi/1
  Divide/1 -> 4*zeta*pi/1
  Divide1/1 -> pi/zeta/1
  pi/zeta/1 -> pi/(zeta*T_transfer)/s/1
  pi/(zeta*T_transfer)/s/1 -> Sum2/1, For saving position  and velocity until after switchover/1, Data Type Conversion4/1
  4*zeta*pi/T_transfer /s/1 -> Divide1/1, Sum1/2
  Sum1/1 -> Divide/1
  4*zeta*pi/1 -> 4*zeta*pi/T_transfer /s/1
  T/1 -> [T]
  Step IN Reset on  either/1 -> [Step], Sum2/2
  [Step] -> 4*zeta*pi/T_transfer /s/2
  [Step] -> pi/(zeta*T_transfer)/s/2
  [T] -> Divide/2
  For saving position  and velocity until after switchover/1 -> Discrete Derivative/1, pi/(zeta*T_transfer)/s/3
  [T] -> Product/1
  (zeta*T_transfer)/pi/1 -> 4*zeta*pi/T_transfer /s/3
  [T] -> Divide1/2
  Sum2/1 -> Sum1/1
  Data Type Conversion4/1 -> Out/1

== system M37_Sim_Forcing_003h_expe_infra_transz_lim/Breaking_Control 20/07/15/Ellipse motion/Phase Shifted Sine 17th 2015/Smooth Displacement Second-Order Filter, zeta 0.8 ==
  note: s
  note: m
  note: y
  note: p
  note: t
  Step IN Reset on  either : Inport
  T : Inport  Port=2  OutDataType=fixdt(1, 16)  OutScaling=2^0
  (zeta*T_transfer)/pi : Gain  Gain=0.8/pi  ParameterDataType=fixdt(1, 16)  ParameterScaling=2^0  OutDataType=fixdt(1, 16)  OutScaling=2^0
  4*zeta*pi : Gain  Gain=3.2*pi  ParameterDataType=fixdt(1, 16)  ParameterScaling=2^0  OutDataType=fixdt(1, 16)  OutScaling=2^0
  4*zeta*pi/T_transfer /s : DiscreteIntegrator  gainval=1  ExternalReset=either  InitialConditionSource=external  SampleTime=-1  OutDataType=fixdt(1, 16)  OutScaling=2^0  ICPrevOutput=DiscIntNeverNeededParam  ICPrevScaledInput=DiscIntNeverNeededParam
  Data Type Conversion4 : DataTypeConversion  OutDataTypeMode=single  OutDataType=fixdt(1, 16)  OutScaling=2^0  OutDataTypeStr=single
  Discrete Derivative : simulink/Discrete/Discrete Derivative  SystemSampleTime=-1  gainval=1.0  ICPrevScaledInput=0.0  OutMin=[]  OutMax=[]  OutDataType=fixdt(1, 16)  OutScaling=2^-10  DoSatur=off
  Divide : Product  Inputs=*/  OutDataType=fixdt(1, 16)  OutScaling=2^-10
  Divide1 : Product  Inputs=*/  OutDataType=fixdt(1, 16)  OutScaling=2^-10
  For saving position  and velocity until after switchover : UnitDelay  SampleTime=-1
  Product : Product  OutDataType=fixdt(1, 16)  OutScaling=2^0  RndMeth=Zero
  Sum1 : Sum  Inputs=|+-  OutDataType=fixdt(1, 16)  OutScaling=2^0
  Sum2 : Sum  Inputs=-+|  OutDataType=fixdt(1, 16)  OutScaling=2^0
  pi/(zeta*T_transfer)/s : DiscreteIntegrator  gainval=1  ExternalReset=either  InitialConditionSource=external  SampleTime=-1  OutDataType=fixdt(1, 16)  OutScaling=2^0  ICPrevOutput=DiscIntNeverNeededParam  ICPrevScaledInput=DiscIntNeverNeededParam
  pi/zeta : Gain  Gain=pi/0.8  ParameterDataType=fixdt(1, 16)  ParameterScaling=2^0  OutDataType=fixdt(1, 16)  OutScaling=2^0
  Out : Outport
  wires:
  Discrete Derivative/1 -> Product/2
  Product/1 -> (zeta*T_transfer)/pi/1
  Divide/1 -> 4*zeta*pi/1
  Divide1/1 -> pi/zeta/1
  pi/zeta/1 -> pi/(zeta*T_transfer)/s/1
  pi/(zeta*T_transfer)/s/1 -> Sum2/1, For saving position  and velocity until after switchover/1, Data Type Conversion4/1
  4*zeta*pi/T_transfer /s/1 -> Divide1/1, Sum1/2
  Sum1/1 -> Divide/1
  4*zeta*pi/1 -> 4*zeta*pi/T_transfer /s/1
  T/1 -> [T]
  Step IN Reset on  either/1 -> [Step], Sum2/2
  [Step] -> 4*zeta*pi/T_transfer /s/2
  [Step] -> pi/(zeta*T_transfer)/s/2
  [T] -> Divide/2
  For saving position  and velocity until after switchover/1 -> Discrete Derivative/1, pi/(zeta*T_transfer)/s/3
  [T] -> Product/1
  (zeta*T_transfer)/pi/1 -> 4*zeta*pi/T_transfer /s/3
  [T] -> Divide1/2
  Sum2/1 -> Sum1/1
  Data Type Conversion4/1 -> Out/1

== system M37_Sim_Forcing_003h_expe_infra_transz_lim/Breaking_Control 20/07/15/Move_cabin/expe_phase/Rate Control Dynamics X ==
  X_vel (cm/sec) : Inport
  trigger : Inport  Port=2
  reset : Inport  Port=3
  stim_X (cm/s) : Inport  Port=4
  zeroing_time : Inport  Port=5
  Constant : Constant  Value=0.2  OutDataType=fixdt(1, 16)  OutScaling=2^0
  Constant1 : Constant  Value=15  OutDataType=fixdt(1, 16)  OutScaling=2^0
  Constant2 : Constant  Value=0.1  OutDataType=fixdt(1, 16)  OutScaling=2^0
  Discrete-Time Integrator1 : DiscreteIntegrator  ExternalReset=either  SampleTime=0.004  OutDataType=fixdt(1, 16)  OutScaling=2^0  ICPrevOutput=DiscIntNeverNeededParam  ICPrevScaledInput=DiscIntNeverNeededParam
  Display1 : Display
  Display2 : Display
  Display4 : Display
  Product : Product  OutDataType=fixdt(1, 16)  OutScaling=2^0  RndMeth=Zero
  "Second-Order Filter, zeta 0.8" : Subsystem
  "Smooth Displacement Second-Order Filter, zeta 0.8" : Subsystem
  Sum2 : Sum  Inputs=++|  OutDataType=fixdt(1, 16)  OutScaling=2^0
  Switch : Switch  Criteria=u2 > Threshold  OutDataType=fixdt(1, 16)  OutScaling=2^0
  X (cm) : Outport
  wires:
  "Second-Order Filter, zeta 0.8"/1(x) -> Discrete-Time Integrator1/1
  Constant/1 -> "Second-Order Filter, zeta 0.8"/2(T)
  Discrete-Time Integrator1/1 -> Product/1, Display2/1
  Product/1 -> X (cm)/1
  "Smooth Displacement Second-Order Filter, zeta 0.8"/1(Out) -> Product/2, Display4/1
  reset/1 -> Discrete-Time Integrator1/2
  trigger/1 -> "Smooth Displacement Second-Order Filter, zeta 0.8"/1(Step IN Reset on  either), Switch/2
  Switch/1 -> "Smooth Displacement Second-Order Filter, zeta 0.8"/2(T)
  Constant2/1 -> Switch/1
  stim_X (cm/s)/1 -> Sum2/1, Display1/1
  zeroing_time/1 -> Switch/3
  Sum2/1 -> "Second-Order Filter, zeta 0.8"/1(u)
  X_vel (cm/sec)/1 -> Sum2/2

== system M37_Sim_Forcing_003h_expe_infra_transz_lim/Breaking_Control 20/07/15/Move_cabin/expe_phase/Rate Control Dynamics Y ==
  Y_vel (cm/sec) : Inport
  trigger : Inport  Port=2
  reset : Inport  Port=3
  stim_Y : Inport  Port=4
  zeroing_time : Inport  Port=5
  Constant : Constant  Value=0.2  OutDataType=fixdt(1, 16)  OutScaling=2^0
  Constant1 : Constant  Value=15  OutDataType=fixdt(1, 16)  OutScaling=2^0
  Constant3 : Constant  Value=0.1  OutDataType=fixdt(1, 16)  OutScaling=2^0
  Discrete-Time Integrator1 : DiscreteIntegrator  ExternalReset=either  SampleTime=0.004  OutDataType=fixdt(1, 16)  OutScaling=2^0  ICPrevOutput=DiscIntNeverNeededParam  ICPrevScaledInput=DiscIntNeverNeededParam
  Display4 : Display
  Product : Product  OutDataType=fixdt(1, 16)  OutScaling=2^0  RndMeth=Zero
  "Second-Order Filter, zeta 0.8" : Subsystem
  "Smooth Displacement Second-Order Filter, zeta 0.8" : Subsystem
  Sum2 : Sum  Inputs=++|  OutDataType=fixdt(1, 16)  OutScaling=2^0
  Switch : Switch  Criteria=u2 > Threshold  OutDataType=fixdt(1, 16)  OutScaling=2^0
  Y (cm) : Outport
  wires:
  "Second-Order Filter, zeta 0.8"/1(x) -> Discrete-Time Integrator1/1
  Constant/1 -> "Second-Order Filter, zeta 0.8"/2(T)
  Discrete-Time Integrator1/1 -> Product/1
  Product/1 -> Y (cm)/1
  "Smooth Displacement Second-Order Filter, zeta 0.8"/1(Out) -> Product/2, Display4/1
  trigger/1 -> "Smooth Displacement Second-Order Filter, zeta 0.8"/1(Step IN Reset on  either), Switch/2
  reset/1 -> Discrete-Time Integrator1/2
  Constant3/1 -> Switch/1
  Switch/1 -> "Smooth Displacement Second-Order Filter, zeta 0.8"/2(T)
  stim_Y/1 -> Sum2/1
  zeroing_time/1 -> Switch/3
  Sum2/1 -> "Second-Order Filter, zeta 0.8"/1(u)
  Y_vel (cm/sec)/1 -> Sum2/2

== system M37_Sim_Forcing_003h_expe_infra_transz_lim/Breaking_Control 20/07/15/Move_cabin/expe_phase/Rate Control Dynamics Z ==
  Z_vel (cm/sec) : Inport
  trigger : Inport  Port=2
  reset : Inport  Port=3
  stim_Z : Inport  Port=4
  zeroing_time : Inport  Port=5
  Constant : Constant  Value=0.2  OutDataType=fixdt(1, 16)  OutScaling=2^0
  Constant1 : Constant  Value=15  OutDataType=fixdt(1, 16)  OutScaling=2^0
  Constant3 : Constant  Value=0.1  OutDataType=fixdt(1, 16)  OutScaling=2^0
  Discrete-Time Integrator1 : DiscreteIntegrator  ExternalReset=either  SampleTime=0.004  OutDataType=fixdt(1, 16)  OutScaling=2^0  ICPrevOutput=DiscIntNeverNeededParam  ICPrevScaledInput=DiscIntNeverNeededParam
  Display4 : Display
  Product : Product  OutDataType=fixdt(1, 16)  OutScaling=2^0  RndMeth=Zero
  "Second-Order Filter, zeta 0.8" : Subsystem
  "Smooth Displacement Second-Order Filter, zeta 0.8" : Subsystem
  Sum2 : Sum  Inputs=++|  OutDataType=fixdt(1, 16)  OutScaling=2^0
  Switch : Switch  Criteria=u2 > Threshold  OutDataType=fixdt(1, 16)  OutScaling=2^0
  Z (cm) : Outport
  wires:
  "Second-Order Filter, zeta 0.8"/1(x) -> Discrete-Time Integrator1/1
  Constant/1 -> "Second-Order Filter, zeta 0.8"/2(T)
  Discrete-Time Integrator1/1 -> Product/1
  Product/1 -> Z (cm)/1
  "Smooth Displacement Second-Order Filter, zeta 0.8"/1(Out) -> Product/2, Display4/1
  trigger/1 -> "Smooth Displacement Second-Order Filter, zeta 0.8"/1(Step IN Reset on  either), Switch/2
  reset/1 -> Discrete-Time Integrator1/2
  Constant3/1 -> Switch/1
  Switch/1 -> "Smooth Displacement Second-Order Filter, zeta 0.8"/2(T)
  stim_Z/1 -> Sum2/1
  zeroing_time/1 -> Switch/3
  Sum2/1 -> "Second-Order Filter, zeta 0.8"/1(u)
  Z_vel (cm/sec)/1 -> Sum2/2

== system M37_Sim_Forcing_003h_expe_infra_transz_lim/Breaking_Control 20/07/15/Move_cabin/expe_phase/Second-Order Filter, zeta 0.9 ==
  u : Inport
  T : Inport  Port=2  OutDataType=fixdt(1, 16)  OutScaling=2^0
  4*zeta*pi : Gain  Gain=3.6*pi  ParameterDataType=fixdt(1, 16)  ParameterScaling=2^0  OutDataTypeMode=double  OutDataType=fixdt(1, 16)  OutScaling=2^0  OutDataTypeStr=double
  4*zeta*pi/T_transfer /s : DiscreteIntegrator  gainval=1  SampleTime=0.004  OutDataType=fixdt(1, 16)  OutScaling=2^0  ICPrevOutput=DiscIntNeverNeededParam  ICPrevScaledInput=DiscIntNeverNeededParam
  Divide : Product  Inputs=*/  OutDataType=fixdt(1, 16)  OutScaling=2^-10
  Divide1 : Product  Inputs=*/  OutDataType=fixdt(1, 16)  OutScaling=2^-10
  Sum1 : Sum  Inputs=|+-  OutDataType=fixdt(1, 16)  OutScaling=2^0
  Sum2 : Sum  Inputs=-+|  OutDataType=fixdt(1, 16)  OutScaling=2^0
  pi/(zeta*T_transfer)/s : DiscreteIntegrator  gainval=1  SampleTime=0.004  OutDataType=fixdt(1, 16)  OutScaling=2^0  ICPrevOutput=DiscIntNeverNeededParam  ICPrevScaledInput=DiscIntNeverNeededParam
  pi/zeta : Gain  Gain=pi/0.9  ParameterDataType=fixdt(1, 16)  ParameterScaling=2^0  OutDataType=fixdt(1, 16)  OutScaling=2^0
  x : Outport
  wires:
  Divide/1 -> 4*zeta*pi/1
  Divide1/1 -> pi/zeta/1
  pi/zeta/1 -> pi/(zeta*T_transfer)/s/1
  pi/(zeta*T_transfer)/s/1 -> Sum2/1, x/1
  4*zeta*pi/T_transfer /s/1 -> Divide1/1, Sum1/2
  Sum1/1 -> Divide/1
  4*zeta*pi/1 -> 4*zeta*pi/T_transfer /s/1
  T/1 -> [T]
  [T] -> Divide/2
  [T] -> Divide1/2
  Sum2/1 -> Sum1/1
  u/1 -> Sum2/2

== system M37_Sim_Forcing_003h_expe_infra_transz_lim/Breaking_Control 20/07/15/Move_cabin/expe_phase/Stay within ellipse 20/07/15 ==
  x_in (cm) : Inport
  y_in (cm) : Inport  Port=2
  X_size (cm) : Inport  Port=3
  Y_size (cm) : Inport  Port=4
  Alpha : Product  Inputs=*/  OutDataType=fixdt(1, 16)  OutScaling=2^-10
  Constant : Constant  OutDataType=fixdt(1, 16)  OutScaling=2^0
  Divide : Product  Inputs=*/  OutDataType=fixdt(1, 16)  OutScaling=2^-10
  Divide1 : Product  Inputs=*/  OutDataType=fixdt(1, 16)  OutScaling=2^-10
  Divide2 : Product  Inputs=*/  OutDataType=fixdt(1, 16)  OutScaling=2^-10
  Get R : Stateflow chart
  Product : Product  OutDataType=fixdt(1, 16)  OutScaling=2^0  RndMeth=Zero
  Switch : Switch  Threshold=1  OutDataType=fixdt(1, 16)  OutScaling=2^0
  x_out (cm) : Outport
  y_out (cm) : Outport  Port=2
  wires:
  x_in (cm)/1 -> Get R/1(x), Divide1/1
  y_in (cm)/1 -> Divide2/1, Product/1
  Get R/1(R) -> Divide/1
  X_size (cm)/1 -> Divide/2, Alpha/1
  Divide/1 -> Switch/2, Switch/1
  Constant/1 -> Switch/3
  Switch/1 -> Divide1/2, Divide2/2
  Divide1/1 -> x_out (cm)/1
  Divide2/1 -> y_out (cm)/1
  Y_size (cm)/1 -> Alpha/2
  Product/1 -> Get R/2(y)
  Alpha/1 -> Product/2

== system M37_Sim_Forcing_003h_expe_infra_transz_lim/Joint Controller (May 7, 2015)1/Inverse Kinematics May 6, 2015/Inverse Kinematics/full inverse kin ==
  vec : Inport
  Enable : EnablePort
  Embedded MATLAB Function : Stateflow chart
  out : Outport  OutDataType=fixdt(1, 16)  OutScaling=2^0
  wires:
  vec/1 -> Embedded MATLAB Function/1(vec)
  Embedded MATLAB Function/1(out) -> out/1

== system M37_Sim_Forcing_003h_expe_infra_transz_lim/Joint Controller (May 7, 2015)1/Inverse Kinematics May 6, 2015/Simplified Inverse Kinematics/A1-A6 COM ==
  vec : Inport
  Demux1 : Demux  Outputs=7
  Ground : Ground
  Ground1 : Ground
  Ground2 : Ground
  Mux1 : Mux  Inputs=6
  Terminator{,1..3} (4 alike) : Terminator
  A1-A6 COM : Outport
  wires:
  Demux1/2 -> Mux1/2
  Demux1/3 -> Mux1/3
  Demux1/5 -> Mux1/5
  Ground/1 -> Mux1/1
  Ground1/1 -> Mux1/4
  Ground2/1 -> Mux1/6
  Demux1/1 -> Terminator/1
  Demux1/4 -> Terminator1/1
  Demux1/6 -> Terminator2/1
  Demux1/7 -> Terminator3/1
  Mux1/1 -> A1-A6 COM/1
  vec/1 -> Demux1/1

== system M37_Sim_Forcing_003h_expe_infra_transz_lim/Joint Controller (May 7, 2015)1/Inverse Kinematics May 6, 2015/Simplified Inverse Kinematics/Simplified Inverse Kin ==
  Vec : Inport  OutDataType=fixdt(1, 16)  OutScaling=2^0
  Enable : EnablePort
  Display : Display
  Display1 : Display
  Display2 : Display
  Embedded MATLAB Function1 : Stateflow chart
  Embedded MATLAB Function2 : Stateflow chart
  Embedded MATLAB Function3 : Stateflow chart
  Out : Outport
  Out_MGI : Outport  Port=2
  wires:
  Vec/1 -> Embedded MATLAB Function1/1(vec), Embedded MATLAB Function3/1(vec), Display1/1
  Embedded MATLAB Function1/1(out) -> Out/1
  Embedded MATLAB Function3/1(out) -> Out_MGI/1, Display/1, Embedded MATLAB Function2/1(vec)
  Embedded MATLAB Function2/1(out) -> Display2/1
